simulink model "get_jntTgts_Track"  (R2026a)
settings: Solver=ode23t  AbsTol=1e-3  EnableMultiTasking=on
libraries: fl_lib x4, sm_lib x2, nesl_utility x2, sdl_lib x1, sm_trackV_lib_chain_lower_frame_s46i1u2l7 x1
Description:
  | Copyright 2024-2026 The MathWorks, Inc.
settings Model: Creator=smiller  LastModifiedBy=smiller
settings DebuggingCC: SubsystemReferenceDiagnosticForUnitTest=warning
settings SimscapeCC: SimscapeNominalValues="[{\"value\":\"1\",\"unit\":\"A\"},{\"value\":\"1\",\"unit\":\"bar\"},{\"value\":\"1\",\"unit\":\"cm^2\"},{\"value\":\"1\",\"unit\":\"cm^3/s\"},{\"value\":\"1\",\"unit\":\"kJ/kg\"},{\"value\":\"1\",\"unit\":\"kW\"},{\"value\":\"1\",\"unit\":\"l\"},{\"value\":\"1\",\"unit\":\"N\"},{\"value\":\"1\",\"unit\":\"N*m\"},{\"value\":\"1\",\"unit\":\"V\"}]"  SimscapeLogSimulationStatistics=on  SimscapeLogName=simlog_getChainJointTargets  SimscapeLogLimitData=off
settings DiagnosticsConfigSet: SimMechanicsUnconnectedFramePorts=none  SimMechanicsConflictingReferenceFrames=none
settings ExplorerConfigSet: InternalSimMechanicsExplorerSettings="<ExplorerConfiguration><canonicalview>default</canonicalview><AnimationSetting><BasePlaybackSpeed>1.0</BasePlaybackSpeed><PlaybackSpeedFactor>1.0</PlaybackSpeedFactor></AnimationSetting><TilePanel><TileInfo><Tiles Columns=\"1\" Count=\"1\" Rows=\"1\"><Column Weight=\"1\"/><Row Weight=\"1\"/><Tile Height=\"1\" Width=\"1\" X=\"0\" Y=\"0\"/></Tiles></TileInfo><SceneInfo><SceneViewer><BGColor><R>1</R><G>1</G><B>1</B></BGColor><Camera><DoPerspective>off</DoPerspective><Position><X>1.0675961971282959</X><Y>0.150476992130279652</Y><Z>-2.55170276731864298</Z></Position><Center><X>1.0675961971282959</X><Y>0.150476992130279652</Y><Z>5.80442609532383358e-08</Z></Center><Up><X>0</X><Y>-1</Y><Z>0</Z></Up><ViewLimDist>1</ViewLimDist><YLim>1.88530440198739591</YLim><XLim>2.30492700338363665</XLim></Camera></SceneViewer></SceneInfo></TilePanel><MechEditorPanel><Cameras/><GfxPanelCameraMap/><VideoCreator><PlaybackSpeedRatio>1.0</PlaybackSpeedRatio><FrameRate>30</FrameRate><VideoFormat>Motion JPEG AVI</VideoFormat><FrameSize>auto</FrameSize></VideoCreator></MechEditorPanel></ExplorerConfiguration>"

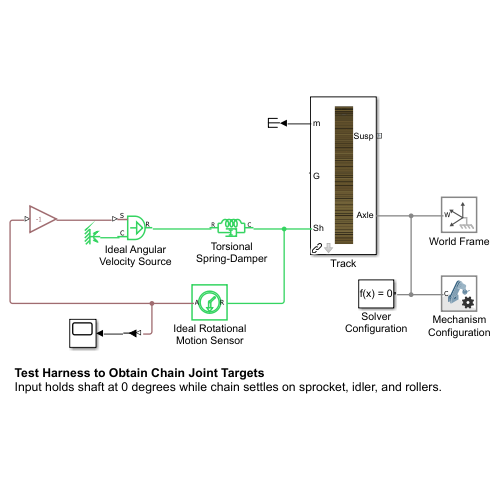
[thumbnail: Simulink's stored preview of the top-level diagram]
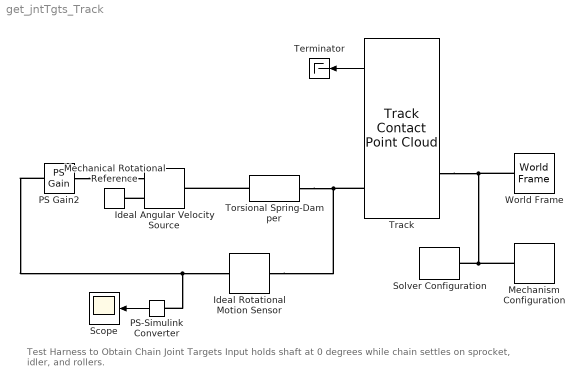
== system get_jntTgts_Track ==
  note: Test Harness to Obtain Chain Joint Targets
      | Input holds shaft at 0 degrees while chain settles on sprocket, idler, and rollers.
  Ideal Angular Velocity Source : fl_lib/Mechanical/Mechanical Sources/Ideal Angular Velocity Source
  Ideal Rotational Motion Sensor : fl_lib/Mechanical/Mechanical Sensors/Ideal Rotational Motion Sensor  reference=foundation.enum.MeasurementReference.absolute  acceleration_port=false  velocity_port=false  position_port=true  wrap_angle=false  offset=0 rad
  Mechanical Rotational Reference : fl_lib/Mechanical/Rotational Elements/Mechanical Rotational Reference
  Mechanism Configuration : sm_lib/Utilities/Mechanism Configuration  UniformGravity=Constant  GravityVector=[0 0 -9.80665]  GravityVectorUnits=m/s^2  LinearizationDelta=0.001  JointModeTransitionNonlinearIterations=2
  PS Gain2 : fl_lib/Physical Signals/Functions/PS Gain  gain=-1 deg/s/deg
  PS-Simulink Converter : nesl_utility/PS-Simulink Converter  PhysicalDomain=network_engine_domain  SubClassName=ps_output  LeftPortType=input  RightPortType=output  PseudoPeriodic=off  Frequencies=[]  VectorFormat=inherit  Unit=inherit  AffineConversion=off
  Scope : Scope
      settings: ActiveDisplayYMinimum=-0.00418  ActiveDisplayYMaximum=0.00056
  Solver Configuration : nesl_utility/Solver Configuration  PhysicalDomain=network_engine_domain  SubClassName=solver  LeftPortType=input  RightPortType=generic  Tones=[]  Harmonics=[]  SimulateNoise=off  Profile=off  UseLocalSampling=off  EnableSwitchedLinearOptims=on  FrequencyDomain=off  UseCCode=off  RelTol=0.001  AbsTol=1e-06  MinStep=1e-09  ToWorkspace=off  RevertToSquareIcSolve=off  NumHomotopyIterations=100  PhasorMode=off  PhasorModeNumHarmonics=1  ConsistencySolver=NEWTON_XTOL_AFTER_FTOL  CanonicalOrdering=UNORDERED  OptimizeIntermediates=UNOPTIMIZED  IndexReductionMethod=DerivativeReplacement  DoDC=off  ResidualTolerance=1e-09  ConsistencyTolSource=GLOBAL  ConsistencyAbsTol=0.001  ConsistencyRelTol=0.001  ConsistencyTolFactor=0.001  UseLocalSolver=off  LocalSolverChoice=NE_BACKWARD_EULER_ADVANCER  ResolveIndetEquations=on  FunctionEvalNumThread=1  LocalSolverSampleTime=0.001  DoFixedCost=off  MaxNonlinIter=3  MaxModeIter=2  ComputeImpulses=off  ImpulseIterations=2  LinearAlgebra=Sparse  LinearAlgebraNumThread=0  EquationFormulation=NE_TIME_EF  DelaysMemoryBudget=1024  AutomaticFiltering=on  FilteringTimeConstant=0.001  PartitionStorageMethod=AS_NEEDED  PartitionMemoryBudget=1024  PartitionMethod=FAST  MultibodyUseLocalSolver=off  MultibodyLocalSolverChoice=ODE1  MultibodyLocalSolverSampleTime=0.001
  Terminator : Terminator
  Torsional Spring-Damper : sdl_lib/Couplings & Drives/Torsional Spring-Damper  k=1e5 N*m/rad  mu_visc=1e4 N*m*s/rad  trq_coulomb=0 N*m  static_kinetic_ratio=1.1  w_tol=0.001 rad/s  model_hardstop=sdl.enum.hardStopOffOn.off  upper_bound=10 deg  lower_bound=-10 deg  hardstop_model=simscape.enum.hardstop.smooth  k_endstop=1e6 N*m/rad  D_endstop=10 N*m*s/rad  transition=0.001 rad  coeff_rest=0.7  w_tol_hardstop=0.1 rad/s  trq_tol=0.001 N*m  x0=0 deg
  Track : sm_trackV_lib_chain_lower_frame_s46i1u2l7/Track Contact Point Cloud  popup_leftOrRight=Left  sprk_xc=Excv.Sprocket.sprocket_xc  sprk_len=Excv.Sprocket.sprk_width  sprk_rho=Excv.Sprocket.density  sprk_clr=Excv.Sprocket.clr  sprk_opc=Excv.Sprocket.opc  sprk_contact_geo_ptcld=Excv.Sprocket.teeth_contact.ptcld.pts  sprk_contact_geo_rad=Excv.Sprocket.teeth_contact.ptcld.rad  sprk_contact_geo_clr=Excv.Sprocket.teeth_contact.ptcld.clr  sprk_contact_geo_opc=Excv.Sprocket.teeth_contact.ptcld.opc  idler_rad=Excv.Idler.rad  idler_len=Excv.Idler.len  idler_rho=Excv.Idler.rho  idler_clr=Excv.Idler.clr  idler_opc=Excv.Idler.opc  idler_contgeo_clr=Excv.Idler.chain_contact.clr  idler_contgeo_opc=Excv.Idler.chain_contact.opc  roller_upper_rad=Excv.Roller.Upper.rad  roller_upper_len=Excv.Roller.Upper.len  roller_upper_rho=Excv.Roller.Upper.rho  roller_upper_clr=Excv.Roller.Upper.clr  roller_upper_opc=Excv.Roller.Upper.opc  roller_upper_contgeo_clr=[1.0 0.0 0.0]  roller_upper_contgeo_opc=1  roller_lower_rad=Excv.Roller.Lower.rad  roller_lower_len=Excv.Roller.Lower.len  roller_lower_rho=Excv.Roller.Lower.rho  roller_lower_clr=Excv.Roller.Lower.clr  roller_lower_opc=Excv.Roller.Lower.opc  roller_lower_contgeo_clr=[1.0 0.0 0.0]  roller_lower_contgeo_opc=1  tensioner_cyl_len=Excv.Idler.Tensioner.cyl.len  tensioner_cyl_rad=Excv.Idler.Tensioner.cyl.rad  tensioner_cyl_rho=Excv.Idler.Tensioner.cyl.rho  tensioner_cyl_clr=Excv.Idler.Tensioner.cyl.clr  tensioner_cyl_opc=Excv.Idler.Tensioner.cyl.opc  tensioner_pist_len=Excv.Idler.Tensioner.piston.len  tensioner_pist_rad=Excv.Idler.Tensioner.piston.rad  tensioner_pist_rho=Excv.Idler.Tensioner.piston.rho  tensioner_pist_clr=Excv.Idler.Tensioner.piston.clr  tensioner_pist_opc=Excv.Idler.Tensioner.piston.opc  tensioner_br_length=Excv.Idler.Tensioner.bracket.len  tensioner_br_width=Excv.Idler.Tensioner.bracket.wid  tensioner_br_height=Excv.Idler.Tensioner.bracket.height  tensioner_br_thk=Excv.Idler.Tensioner.bracket.thk  tensioner_br_rho=Excv.Idler.Tensioner.bracket.rho  tensioner_br_clr=Excv.Idler.Tensioner.bracket.clr  tensioner_br_opc=Excv.Idler.Tensioner.bracket.opc  tensioner_eqpos=Excv.Idler.Tensioner.xeq  tensioner_x0=Excv.Idler.Tensioner.x0  tensioner_k=Excv.Idler.Tensioner.K  tensioner_b=Excv.Idler.Tensioner.B  roller_upper_x=Excv.Frame.Sprk2UpperX  roller_lower_x=Excv.Frame.Sprk2LowerX  idler_x=Excv.Frame.IdlerAssyX  axle_x=Excv.Frame.AxleX  roller_upper_y=Excv.Frame.Sprk2UpperY  roller_lower_y=Excv.Frame.Sprk2LowerY  idler_y=Excv.Frame.Sprk2IdlerY  sprk_pitch_rad=Excv.Sprocket.sprocket_rPitch  axle_y=Excv.Frame.AxleY  frame_cg_offset=Excv.Frame.CGOffset  frame_mass=Excv.Frame.Mass  frame_moi=Excv.Frame.MOI  frame_poi=Excv.Frame.POI  frame_susp_offset=Excv.Frame.SuspOffset  chain_wid=Excv.Chain.chain_wid  chain_seg_m=Excv.Chain.link_m  chain_seg_cg=Excv.Chain.link_cg  chain_seg_moi=Excv.Chain.link_moi  chain_seg_poi=Excv.Chain.link_poi  plate_xc=Excv.Chain.plate_xc  plate_h=Excv.Chain.plate_h  pin_sep=Excv.Chain.pin_sep  plate_thk=Excv.Chain.plate_thk  plate_ang=Excv.Chain.plate_ang  plate_clr=Excv.Chain.plate_clr  plate_opc=Excv.Chain.plate_opc  pin_len=Excv.Chain.pin_len  pin_rad=Excv.Chain.pin_rad  pin_clr=Excv.Chain.pin_clr  pin_opc=Excv.Chain.pin_opc  shoe_xc=Excv.Shoe.xc  shoe_w=Excv.Shoe.w  shoe_m=Excv.Shoe.mass  shoe_cg=Excv.Shoe.cg  shoe_moi=Excv.Shoe.moi  shoe_poi=Excv.Shoe.poi  shoe_clr=Excv.Shoe.clr  shoe_opc=Excv.Shoe.opc  jointTargets=track_joint_targets  chainDamping=Excv.Chain.damping  ptcld_shoe=Excv.Shoe.ground_contact.ptcld.pts  ptcld_shoe_rad=Excv.Shoe.ground_contact.ptcld.rad  ptcld_shoe_clr=Excv.Shoe.ground_contact.ptcld.clr  ptcld_shoe_opc=Excv.Shoe.ground_contact.ptcld.opc  chain_to_roller_clr=Excv.Chain.roller_contact.clr  chain_to_roller_opc=Excv.Chain.roller_contact.opc  chain_to_teeth_clr=Excv.Chain.teeth_contact.clr  chain_to_teeth_opc=Excv.Chain.teeth_contact.opc  B_Sprocket=Excv.Contact.Sprocket.B  K_Sprocket=Excv.Contact.Sprocket.K  TW_Sprocket=Excv.Contact.Sprocket.TW  K_Roller=Excv.Contact.Roller.K  B_Roller=Excv.Contact.Roller.B  TW_Roller=Excv.Contact.Roller.TW  K_Idler=Excv.Contact.Idler.K  B_Idler=Excv.Contact.Idler.B  TW_Idler=Excv.Contact.Idler.TW  popup_sense_roller=Actuator Torque
  World Frame : sm_lib/Frames and Transforms/World Frame
  wires:
  PS-Simulink Converter/1 -> Scope/1
  Track/1 -> Terminator/1
  connections:
  World Frame/RConn1 -- Track/LConn2 -- Mechanism Configuration/RConn1 -- Solver Configuration/RConn1
  Torsional Spring-Damper/LConn1 -- Ideal Angular Velocity Source/LConn1
  Torsional Spring-Damper/RConn1 -- Track/RConn2 -- Ideal Rotational Motion Sensor/LConn1
  Ideal Angular Velocity Source/RConn2 -- Mechanical Rotational Reference/LConn1
  PS Gain2/LConn1 -- PS-Simulink Converter/LConn1 -- Ideal Rotational Motion Sensor/RConn1
  PS Gain2/RConn1 -- Ideal Angular Velocity Source/RConn1
